simulink model "pid"  (Simulink 7.1)
settings: Solver=ode3  StartTime=0.0  StopTime=20  RelTol=1e-3
settings Model: Creator=Administrator  LastModifiedBy=xierthy
settings OptimizationCC: InlineInvariantSignals=on
settings DebuggingCC: SaveWithParameterizedLinksMsg=none  SignalResolutionControl=TryResolveAllWithWarning  MultiTaskDSMMsg=warning  MultiTaskCondExecSysMsg=none  StrictBusMsg=None
settings RTWCC: IncludeERTFirstTime=on
settings GRTTargetCC: TargetFcnLib=ansi_tfl_tmw.mat

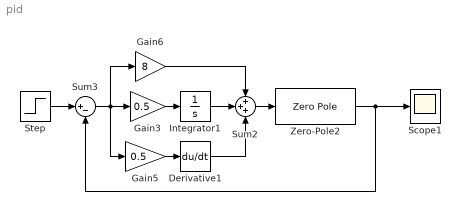
== system pid ==
  Derivative1 : Derivative
  Gain3 : Gain  Gain=0.5  ParameterDataType=sfix(16)  ParameterScaling=2^0  OutDataType=sfix(16)  OutScaling=2^0
  Gain5 : Gain  Gain=0.5  ParameterDataType=sfix(16)  ParameterScaling=2^0  OutDataType=sfix(16)  OutScaling=2^0
  Gain6 : Gain  Gain=8  ParameterDataType=sfix(16)  ParameterScaling=2^0  OutDataType=sfix(16)  OutScaling=2^0
  Integrator1 : Integrator
  Scope1 : Scope
      settings: TimeRange=20  YMin=0.98  YMax=1.07  SaveName=ScopeData2
  Step : Step  Time=0  SampleTime=0
  Sum2 : Sum  Inputs=+++  OutDataType=sfix(16)  OutScaling=2^0
  Sum3 : Sum  Inputs=|+-  OutDataType=sfix(16)  OutScaling=2^0
  Zero-Pole2 : ZeroPole  Zeros=[-0.5]  Poles="[-1  -1 -1]"  Gain=[10]
  wires:
  Sum3/1 -> Gain3/1, Gain5/1, Gain6/1
  Gain5/1 -> Derivative1/1
  Gain3/1 -> Integrator1/1
  Integrator1/1 -> Sum2/2
  Derivative1/1 -> Sum2/3
  Zero-Pole2/1 -> Sum3/2, Scope1/1
  Sum2/1 -> Zero-Pole2/1
  Gain6/1 -> Sum2/1
  Step/1 -> Sum3/1
